simulink model "controllore_es"  (Simulink 8.3)
settings: Solver=ode45  StartTime=0.0  StopTime=20  RelTol=1e-3
values from neighbouring files (symbols this model uses):
  Kr = 1    [controllore.m]
libraries: cstblocks x3
settings Model: Creator=matdo  LastModifiedBy=matdo
settings DataIOCC: SignalLoggingSaveFormat=Dataset
settings DebuggingCC: UnderspecifiedInitializationDetection=Simplified  StateNameClashWarn=none
settings GRTTargetCC: CombineOutputUpdateFcns=on  GRTInterface=off

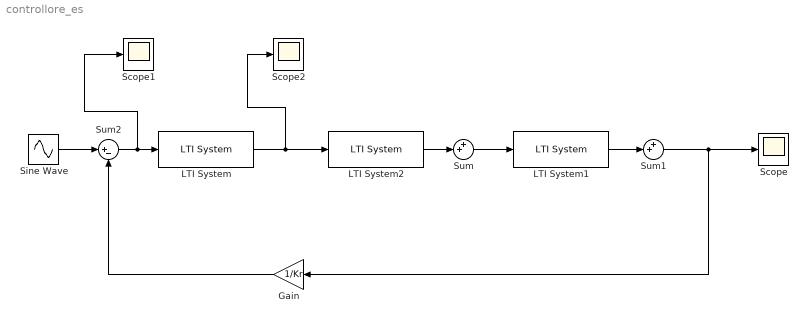
== system controllore_es ==
  Gain : Gain  Gain=1/Kr
  LTI System : cstblocks/LTI System  sys=Ci  IC=[]
  LTI System1 : cstblocks/LTI System  sys=F2  IC=[]
  LTI System2 : cstblocks/LTI System  sys=F1  IC=[]
  Scope : Scope
  Scope1 : Scope
  Scope2 : Scope
      settings: SaveName=ScopeData2
  Sine Wave : Sin  Frequency=0.2  SampleTime=0
  Sum : Sum  Inputs=++|
  Sum1 : Sum  Inputs=++|
  Sum2 : Sum  Inputs=|+-
  wires:
  Gain/1 -> Sum2/2
  Sine Wave/1 -> Sum2/1
  Sum2/1 -> Scope1/1, LTI System/1
  LTI System/1 -> Scope2/1, LTI System2/1
  LTI System2/1 -> Sum/2
  Sum/1 -> LTI System1/1
  LTI System1/1 -> Sum1/2
  Sum1/1 -> Gain/1, Scope/1
